simulink model "Lane_ECG_Monitor_Simulink"  (R2024b)
settings: Solver=VariableStepAuto  StartTime=0.0  StopTime=10  RelTol=1e-3
undefined symbols (not defined in the file): D
libraries: dspsigattribs x1, simulink x1, dspstat3 x1, spsSecondOrderFilterLib x1
settings Model: Creator=Hp  LastModifiedBy=Hp

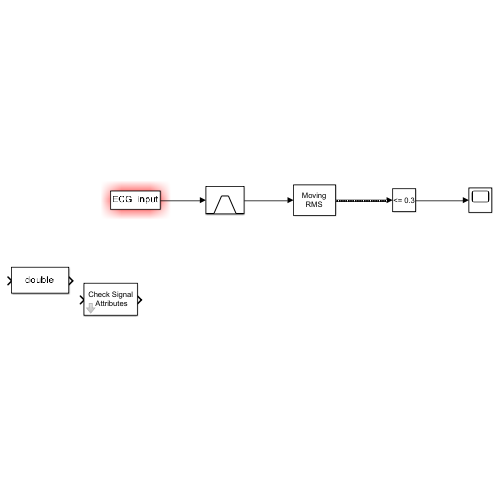
[thumbnail: Simulink's stored preview of the top-level diagram]
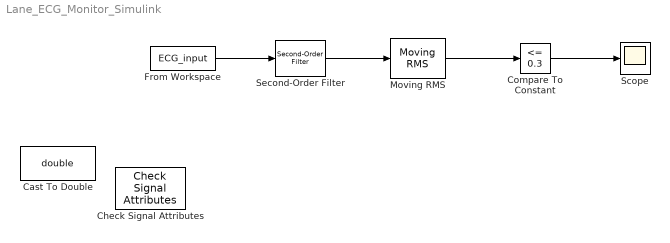
== system Lane_ECG_Monitor_Simulink ==
  Cast To Double : DataTypeConversion  OutDataTypeStr=double  SaturateOnIntegerOverflow=off  RndMeth=Floor
  Check Signal Attributes : dspsigattribs/Check Signal Attributes  SigAttribCheckMethod=Does not match attributes exactly  Complexity=Ignore  Frame=Ignore  DimsCheckMethod=Ignore  Dimensions=1-D  DatatypeCheckMethod=Ignore  DatatypeGeneral=Boolean  DtypeFloatSpecific=Any floating-point  DtypeFixedSpecific=Any fixed-point  DtypeIntSpecific=Any integer  SampleMode=Ignore
  Compare To Constant : simulink/Logic and Bit Operations/Compare To Constant  relop=<=  const=0.3  OutDataTypeStr=boolean
  From Workspace : FromWorkspace  VariableName=ECG_input  SampleTime=-1
  Moving RMS : dspstat3/Moving RMS  Method=Sliding window  ForgettingFactorPort=off  SpecifyWindowLength=on  WindowLength=50  OverlapLength=3  AllowArbitraryInputLength=on  ForgettingFactor=0.9  SimulateUsing=Interpreted execution
  Scope : Scope
  Second-Order Filter : spsSecondOrderFilterLib/Second-Order Filter  FilterType=Bandpass  Fo=4.47  Zeta=0.707  Ts=0.001  Initialize=on  Vac_Init="[0,  0,  60]"  Vdc_Init=0  PlotResponse=off  FreqRange=[0, 500, 1]
      settings: LibrarySourceBlock=|
      | sps_lib/Control/Filters/Second-Order
      | Filter
  wires:
  From Workspace/1 -> Second-Order Filter/1
  Second-Order Filter/1 -> Moving RMS/1
  Moving RMS/1 -> Compare To Constant/1
  Compare To Constant/1 -> Scope/1
